simulink model "static_error_model"  (R2023b)
settings: Solver=FixedStepAuto  StartTime=0.0  StopTime=20000  FixedStep=1e-2  RelTol=1e-3
values from neighbouring files (symbols this model uses):
  A = [-a1, 1 ... (first row only)    [task_1.m]
  A0 = [-k1, 1 ... (first row only)    [task_1.m]
  b = [b1; b0]    [task_1.m]
  C = [1, 0]    [task_1.m]
  D = [0;0]    [task_1.m]
  gamma = 0.5    [task_1.m]
  k0 = 0.64    [task_1.m]
  k1 = 1.6    [task_1.m]
  theta = [k0 - a0 ... (first row only)    [task_1.m]
settings Model: Creator=nguye  LastModifiedBy=nguye

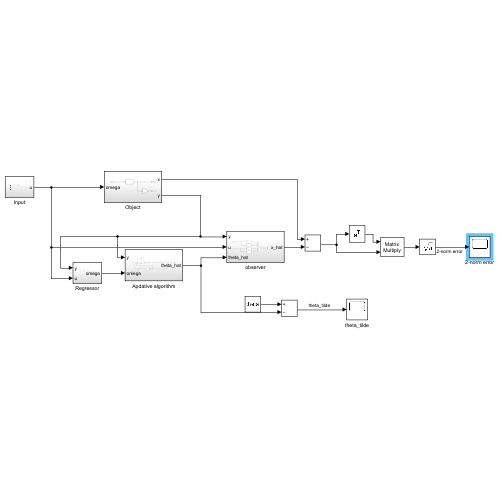
[thumbnail: Simulink's stored preview of the top-level diagram]
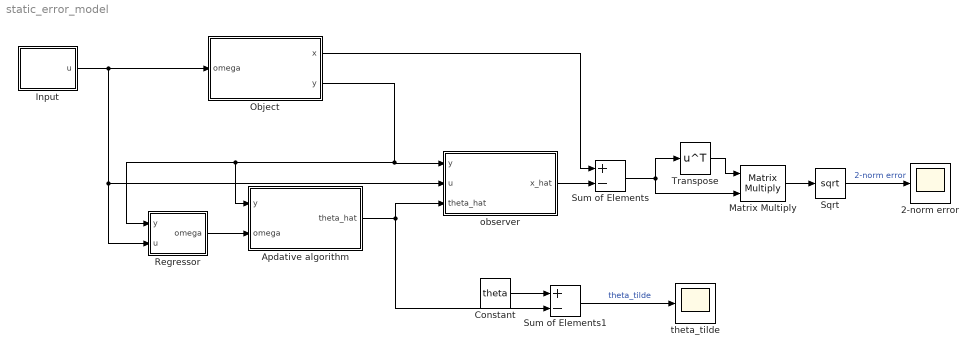
== system static_error_model ==
  2-norm error : Scope
  Apdative algorithm : Subsystem
  Constant : Constant  Value=theta
  Input : Subsystem
  Matrix Multiply : Product  Multiplication=Matrix(*)
  Object : Subsystem
  Regressor : Subsystem
  Sqrt : Sqrt
  Sum of Elements : Sum  Inputs=+-
  Sum of Elements1 : Sum  Inputs=+-
  Transpose : Math  Operator=transpose
  observer : Subsystem
  theta_tilde : Scope
  wires:
  Input/1(u) -> Object/1(omega), observer/2(u), Regressor/2(u)
  Object/2(y) -> observer/1(y), Regressor/1(y), Apdative algorithm/1(y)
  Constant/1 -> Sum of Elements1/1
  Apdative algorithm/1(theta_hat) -> Sum of Elements1/2, observer/3(theta_hat)
  Sum of Elements1/1 -> theta_tilde/1  "theta_tilde"
  Regressor/1(omega) -> Apdative algorithm/2(omega)
  observer/1(x_hat) -> Sum of Elements/2
  Object/1(x) -> Sum of Elements/1
  Matrix Multiply/1 -> Sqrt/1
  Sum of Elements/1 -> Transpose/1, Matrix Multiply/2
  Transpose/1 -> Matrix Multiply/1
  Sqrt/1 -> 2-norm error/1  "2-norm error"

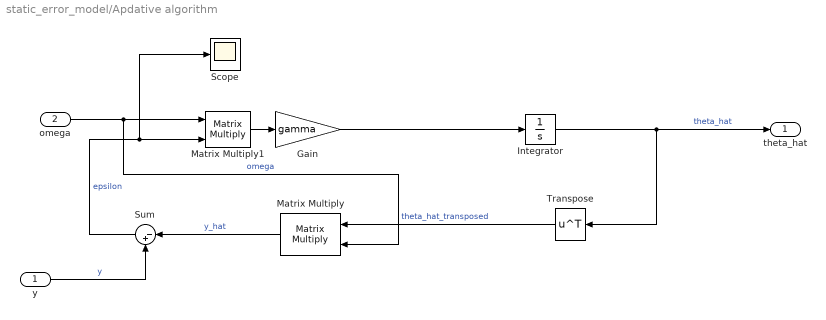
== system static_error_model/Apdative algorithm ==
  y : Inport
  omega : Inport  Port=2
  Gain : Gain  Gain=gamma
  Integrator : Integrator  InitialCondition=[1,1,1,1]
  Matrix Multiply : Product  Multiplication=Matrix(*)
  Matrix Multiply1 : Product  Multiplication=Matrix(*)
  Scope : Scope
  Sum : Sum  Inputs=|-+
  Transpose : Math  Operator=transpose
  theta_hat : Outport
  wires:
  omega/1 -> Matrix Multiply/2, Matrix Multiply1/1  "omega"
  Integrator/1 -> theta_hat/1, Transpose/1  "theta_hat"
  Matrix Multiply/1 -> Sum/1  "y_hat"
  y/1 -> Sum/2  "y"
  Transpose/1 -> Matrix Multiply/1  "theta_hat_transposed"
  Matrix Multiply1/1 -> Gain/1
  Sum/1 -> Scope/1, Matrix Multiply1/2  "epsilon"
  Gain/1 -> Integrator/1

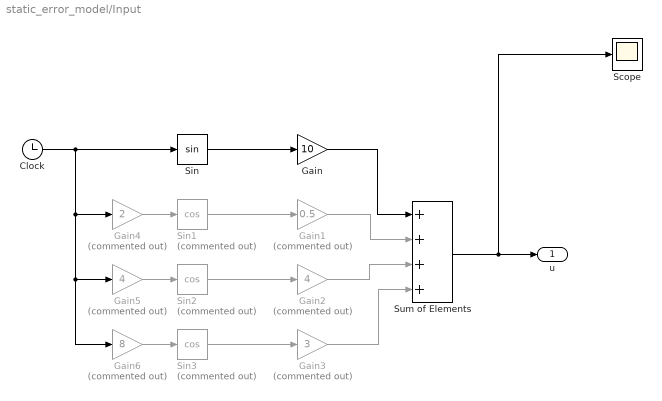
== system static_error_model/Input ==
  Clock : Clock
  Gain : Gain  Gain=10
  Gain1 : Gain  Commented=on  Gain=0.5
  Gain2 : Gain  Commented=on  Gain=4
  Gain3 : Gain  Commented=on  Gain=3
  Gain4 : Gain  Commented=on  Gain=2
  Gain5 : Gain  Commented=on  Gain=4
  Gain6 : Gain  Commented=on  Gain=8
  Scope : Scope
  Sin : Trigonometry
  Sin1 : Trigonometry  Commented=on  Operator=cos
  Sin2 : Trigonometry  Commented=on  Operator=cos
  Sin3 : Trigonometry  Commented=on  Operator=cos
  Sum of Elements : Sum  Inputs=++++
  u : Outport
  wires:
  Clock/1 -> Gain6/1, Gain5/1, Gain4/1, Sin/1
  Sin/1 -> Gain/1
  Gain/1 -> Sum of Elements/1
  Gain4/1 -> Sin1/1
  Gain5/1 -> Sin2/1
  Gain6/1 -> Sin3/1
  Sin3/1 -> Gain3/1
  Sin2/1 -> Gain2/1
  Sin1/1 -> Gain1/1
  Gain1/1 -> Sum of Elements/2
  Gain2/1 -> Sum of Elements/3
  Gain3/1 -> Sum of Elements/4
  Sum of Elements/1 -> Scope/1, u/1

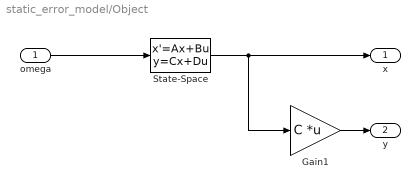
== system static_error_model/Object ==
  omega : Inport
  Gain1 : Gain  Gain=C  Multiplication=Matrix(K*u)
  State-Space : StateSpace  A=A  B=b  C=eye(2)  D=D  InitialCondition=[1, 1]
  x : Outport
  y : Outport  Port=2
  wires:
  omega/1 -> State-Space/1
  State-Space/1 -> Gain1/1, x/1
  Gain1/1 -> y/1

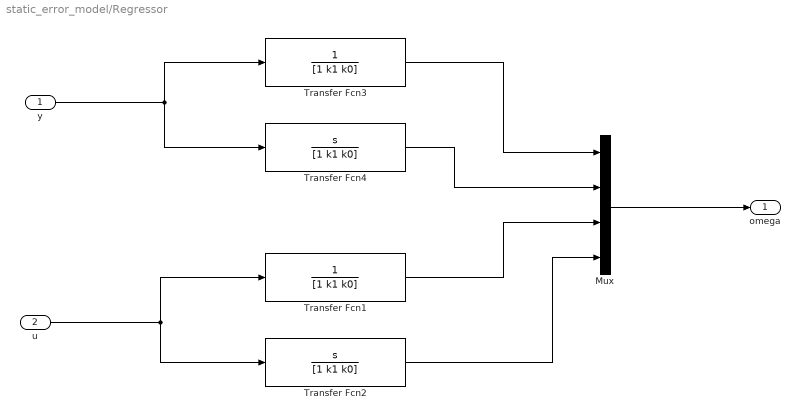
== system static_error_model/Regressor ==
  y : Inport
  u : Inport  Port=2
  Mux : Mux
  Transfer Fcn1 : TransferFcn  Denominator=[1 k1 k0]
  Transfer Fcn2 : TransferFcn  Numerator=[1 0]  Denominator=[1 k1 k0]
  Transfer Fcn3 : TransferFcn  Denominator=[1 k1 k0]
  Transfer Fcn4 : TransferFcn  Numerator=[1 0]  Denominator=[1 k1 k0]
  omega : Outport
  wires:
  y/1 -> Transfer Fcn4/1, Transfer Fcn3/1
  u/1 -> Transfer Fcn1/1, Transfer Fcn2/1
  Transfer Fcn3/1 -> Mux/1
  Transfer Fcn4/1 -> Mux/2
  Transfer Fcn1/1 -> Mux/3
  Transfer Fcn2/1 -> Mux/4
  Mux/1 -> omega/1

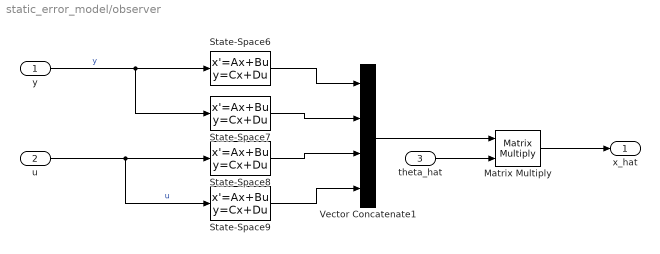
== system static_error_model/observer ==
  y : Inport
  u : Inport  Port=2
  theta_hat : Inport  Port=3
  Matrix Multiply : Product  Multiplication=Matrix(*)
  State-Space6 : StateSpace  A=A0  B=[0;1]  C=eye(2)  D=[0; 0]  InitialCondition=0
  State-Space7 : StateSpace  A=A0  B=[1;0]  C=eye(2)  D=[0; 0]  InitialCondition=0
  State-Space8 : StateSpace  A=A0  B=[0;1]  C=eye(2)  D=[0; 0]  InitialCondition=0
  State-Space9 : StateSpace  A=A0  B=[1;0]  C=eye(2)  D=[0; 0]  InitialCondition=0
  Vector Concatenate1 : Concatenate  NumInputs=4  Mode=Multidimensional array  ConcatenateDimension=2
  x_hat : Outport
  wires:
  y/1 -> State-Space7/1, State-Space6/1  "y"
  u/1 -> State-Space9/1, State-Space8/1  "u"
  State-Space6/1 -> Vector Concatenate1/1
  State-Space7/1 -> Vector Concatenate1/2
  State-Space8/1 -> Vector Concatenate1/3
  State-Space9/1 -> Vector Concatenate1/4
  Vector Concatenate1/1 -> Matrix Multiply/1
  theta_hat/1 -> Matrix Multiply/2
  Matrix Multiply/1 -> x_hat/1
